simulink model "pha_0_5_servovalve"  (R2023a)
settings: Solver=VariableStepAuto  StartTime=0.0  StopTime=15  RelTol=1e-3
libraries: fl_lib x82, SimscapeFluids_lib x26, nesl_utility x8
(part 2 of 2)

== system pha_0_5_servovalve/Servovalve1/Nozzle B ==
  Nozzle B : SimscapeFluids_lib/Isothermal Liquid/Valves & Orifices/Orifices/Orifice (IL)  Tag=Factory Generic  orifice_type=foundation.enum.constant_variable.variable  constant_orifice_spec=fluids.isothermal_liquid.valves_orifices.orifices.enum.constant_orifice_spec.area  variable_orifice_spec=1  orifice_area_constant=1e-3 m^2  p_diff_TLU_constant=[-4, -3, -2, -1, -.5, 0, .5, 1, 2, 3, 4] MPa  vol_flow_TLU_constant=[-2.44, -2.12, -1.68, -1.22, -.84, 0, .85, 1.21, 1.7, 2.09, 2.41] .* 1e-3 m^3/s  S_min=2.9981e-07 m^2/mm  del_S=5.9981e-07 m^2/mm  open_orientation=-1  area_max=3.14 mm^2  area_leak=1e-9 m^2  S_TLU="-([  -0.002 0 0.005 0.015 ]) + 0.001*(0.3) m"  orifice_area_TLU="[  1e-12 4e-12 1e-05 1.02e-05 ] m^2"  area=inf m^2  Cd=0.7  Re_c=150  smoothing_factor=0  pressure_recovery=false  S_vol_flow_TLU="-([  -0.002 0 0.005 0.015 ]) + 0.001*(0.3) m"  p_diff_TLU="[  -5e+06 -2e+06 2e+06 5e+06 ] Pa"  vol_flow_TLU="[  -1e-12 -6e-14 6e+12 1e+11 ; -8e-08 -4e-08 4e+06 8e+06 ; -0.0025 -0.00103 0.001 0.0024 ; -0.00258 -0.001032 0.00106 0.00247 ; ] m^3/s"  enable_faults=simscape.enum.onoff.off  fault_action=fluids.enum.FaultOpening.Closed  external_fault=fluids.enum.FaultExternalTrigger.Off  temporal_fault=simscape.enum.onoff.off  fault_time=5 s  report_fault=simscape.enum.assert.action.none
      settings: InternalSimscapePortConfiguration="{\"Bottom\":[],\"Left\":[{\"id\":\"A\",\"label\":\"A\",\"type\":\"foundation.isothermal_liquid.isothermal_liquid\"},{\"id\":\"S\",\"label\":\"S\",\"type\":\"input\"}],\"Right\":[{\"id\":\"B\",\"label\":\"B\",\"type\":\"foundation.isothermal_liquid.isothermal_liquid\"}],\"Top\":[]}"
  S : PMIOPort  Side=Left
  A : PMIOPort  Port=2  Side=Left
  B : PMIOPort  Port=3  Side=Right
  connections:
  A/RConn1 -- Nozzle B/LConn1
  S/RConn1 -- Nozzle B/LConn2
  B/RConn1 -- Nozzle B/RConn1

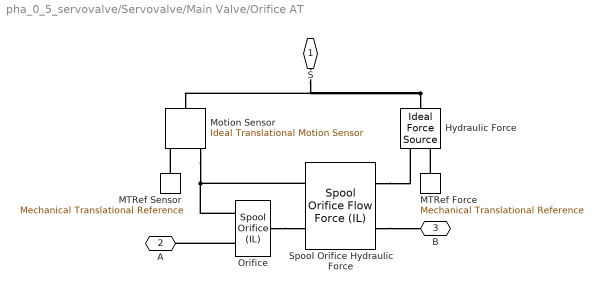
== system pha_0_5_servovalve/Servovalve/Main Valve/Orifice AT ==
  Hydraulic Force : fl_lib/Mechanical/Mechanical Sources/Ideal Force Source  Tag=Factory Generic
  MTRef Force : fl_lib/Mechanical/Translational Elements/Mechanical Translational Reference  Tag=Factory Generic
  MTRef Sensor : fl_lib/Mechanical/Translational Elements/Mechanical Translational Reference  Tag=Factory Generic
  Motion Sensor : fl_lib/Mechanical/Mechanical Sensors/Ideal Translational Motion Sensor  Tag=Factory Generic  reference=foundation.enum.MeasurementReference.difference  acceleration_port=false  velocity_port=true  position_port=true  offset=0 m
  Orifice : SimscapeFluids_lib/Isothermal Liquid/Valves & Orifices/Orifices/Spool Orifice (IL)  Tag=Factory Generic  orifice_spec=2  diameter_hole=5e-3 m  num_hole=6  width=24.5 mm  del_S_max=1 m  S_min=0.01 mm  open_orientation=-1  flow_force_spec=false  clearance=1e-5 m  area_leak=1e-9 m^2  area=inf m^2  Cd=0.7  Re_c=150  smoothing_factor=0  pressure_recovery=false
      settings: InternalSimscapePortConfiguration="{\"Bottom\":[],\"Left\":[{\"id\":\"S\",\"label\":\"S\",\"type\":\"input\"},{\"id\":\"A\",\"label\":\"A\",\"type\":\"foundation.isothermal_liquid.isothermal_liquid\"}],\"Right\":[{\"id\":\"B\",\"label\":\"B\",\"type\":\"foundation.isothermal_liquid.isothermal_liquid\"}],\"Top\":[]}"
  Spool Orifice Hydraulic Force : SimscapeFluids_lib/Isothermal Liquid/Valves & Orifices/Valve Actuators & Forces/Spool Orifice Flow Force (IL)  orifice_spec=2  diameter_hole=0.005 m  num_hole=4  width=24.5 mm  del_S_max=1 m  S_min=0.01 mm  open_orientation=-1  clearance=0.05 mm  area_leak=(24.5)*(0.05) mm^2  smoothing_factor=0
      settings: LibrarySourceBlock=SimscapeFluids_lib/Isothermal Liquid/Valves & Orifices/Valve Actuators & Forces/Spool Orifice Flow Force (IL)  InternalSimscapePortConfiguration="{\"Bottom\":[],\"Left\":[{\"id\":\"A\",\"label\":\"A\",\"type\":\"foundation.isothermal_liquid.isothermal_liquid\"},{\"id\":\"S\",\"label\":\"S\",\"type\":\"input\"}],\"Right\":[{\"id\":\"B\",\"label\":\"B\",\"type\":\"foundation.isothermal_liquid.isothermal_liquid\"},{\"id\":\"F\",\"label\":\"F\",\"type\":\"output\"}],\"Top\":[]}"
  S : PMIOPort  Side=Left
  A : PMIOPort  Port=2  Side=Left
  B : PMIOPort  Port=3  Side=Right
  connections:
  Motion Sensor/RConn3 -- Orifice/LConn1 -- Spool Orifice Hydraulic Force/LConn2
  Hydraulic Force/LConn1 -- Motion Sensor/LConn1 -- S/RConn1
  Orifice/RConn1 -- Spool Orifice Hydraulic Force/LConn1
  Orifice/LConn2 -- A/RConn1
  MTRef Force/LConn1 -- Hydraulic Force/RConn2
  MTRef Sensor/LConn1 -- Motion Sensor/RConn1
  Spool Orifice Hydraulic Force/RConn2 -- Hydraulic Force/RConn1
  Spool Orifice Hydraulic Force/RConn1 -- B/RConn1

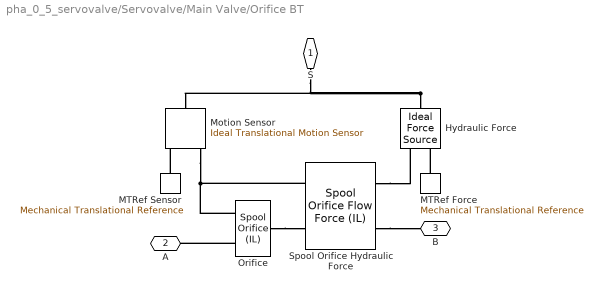
== system pha_0_5_servovalve/Servovalve/Main Valve/Orifice BT ==
  Hydraulic Force : fl_lib/Mechanical/Mechanical Sources/Ideal Force Source  Tag=Factory Generic
  MTRef Force : fl_lib/Mechanical/Translational Elements/Mechanical Translational Reference  Tag=Factory Generic
  MTRef Sensor : fl_lib/Mechanical/Translational Elements/Mechanical Translational Reference  Tag=Factory Generic
  Motion Sensor : fl_lib/Mechanical/Mechanical Sensors/Ideal Translational Motion Sensor  Tag=Factory Generic  reference=foundation.enum.MeasurementReference.difference  acceleration_port=false  velocity_port=true  position_port=true  offset=0 m
  Orifice : SimscapeFluids_lib/Isothermal Liquid/Valves & Orifices/Orifices/Spool Orifice (IL)  Tag=Factory Generic  orifice_spec=2  diameter_hole=5e-3 m  num_hole=6  width=24.5 mm  del_S_max=1 m  S_min=-(0.01) mm  open_orientation=1  flow_force_spec=false  clearance=1e-5 m  area_leak=1e-9 m^2  area=inf m^2  Cd=0.7  Re_c=150  smoothing_factor=0  pressure_recovery=false
      settings: InternalSimscapePortConfiguration="{\"Bottom\":[],\"Left\":[{\"id\":\"S\",\"label\":\"S\",\"type\":\"input\"},{\"id\":\"A\",\"label\":\"A\",\"type\":\"foundation.isothermal_liquid.isothermal_liquid\"}],\"Right\":[{\"id\":\"B\",\"label\":\"B\",\"type\":\"foundation.isothermal_liquid.isothermal_liquid\"}],\"Top\":[]}"
  Spool Orifice Hydraulic Force : SimscapeFluids_lib/Isothermal Liquid/Valves & Orifices/Valve Actuators & Forces/Spool Orifice Flow Force (IL)  orifice_spec=2  diameter_hole=0.005 m  num_hole=4  width=24.5 mm  del_S_max=1 m  S_min=-(0.01) mm  open_orientation=1  clearance=0.05 mm  area_leak=(24.5)*(0.05) mm^2  smoothing_factor=0
      settings: LibrarySourceBlock=SimscapeFluids_lib/Isothermal Liquid/Valves & Orifices/Valve Actuators & Forces/Spool Orifice Flow Force (IL)  InternalSimscapePortConfiguration="{\"Bottom\":[],\"Left\":[{\"id\":\"A\",\"label\":\"A\",\"type\":\"foundation.isothermal_liquid.isothermal_liquid\"},{\"id\":\"S\",\"label\":\"S\",\"type\":\"input\"}],\"Right\":[{\"id\":\"B\",\"label\":\"B\",\"type\":\"foundation.isothermal_liquid.isothermal_liquid\"},{\"id\":\"F\",\"label\":\"F\",\"type\":\"output\"}],\"Top\":[]}"
  S : PMIOPort  Side=Left
  A : PMIOPort  Port=2  Side=Left
  B : PMIOPort  Port=3  Side=Right
  connections:
  Motion Sensor/RConn3 -- Orifice/LConn1 -- Spool Orifice Hydraulic Force/LConn2
  Hydraulic Force/LConn1 -- Motion Sensor/LConn1 -- S/RConn1
  MTRef Sensor/LConn1 -- Motion Sensor/RConn1
  Orifice/LConn2 -- A/RConn1
  MTRef Force/LConn1 -- Hydraulic Force/RConn2
  Spool Orifice Hydraulic Force/RConn1 -- B/RConn1
  Spool Orifice Hydraulic Force/RConn2 -- Hydraulic Force/RConn1
  Orifice/RConn1 -- Spool Orifice Hydraulic Force/LConn1

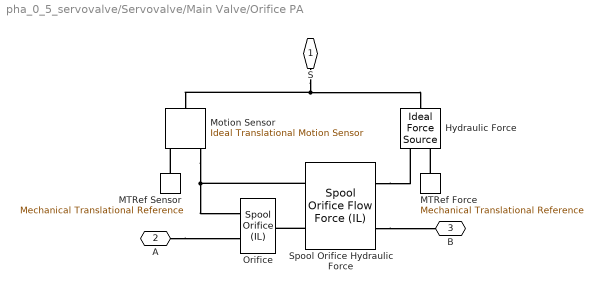
== system pha_0_5_servovalve/Servovalve/Main Valve/Orifice PA ==
  Hydraulic Force : fl_lib/Mechanical/Mechanical Sources/Ideal Force Source  Tag=Factory Generic
  MTRef Force : fl_lib/Mechanical/Translational Elements/Mechanical Translational Reference  Tag=Factory Generic
  MTRef Sensor : fl_lib/Mechanical/Translational Elements/Mechanical Translational Reference  Tag=Factory Generic
  Motion Sensor : fl_lib/Mechanical/Mechanical Sensors/Ideal Translational Motion Sensor  Tag=Factory Generic  reference=foundation.enum.MeasurementReference.difference  acceleration_port=false  velocity_port=true  position_port=true  offset=0 m
  Orifice : SimscapeFluids_lib/Isothermal Liquid/Valves & Orifices/Orifices/Spool Orifice (IL)  Tag=Factory Generic  orifice_spec=2  diameter_hole=5e-3 m  num_hole=6  width=24.5 mm  del_S_max=1 m  S_min=-(0.01) mm  open_orientation=1  flow_force_spec=false  clearance=1e-5 m  area_leak=1e-9 m^2  area=inf m^2  Cd=0.7  Re_c=150  smoothing_factor=0  pressure_recovery=false
      settings: InternalSimscapePortConfiguration="{\"Bottom\":[],\"Left\":[{\"id\":\"S\",\"label\":\"S\",\"type\":\"input\"},{\"id\":\"A\",\"label\":\"A\",\"type\":\"foundation.isothermal_liquid.isothermal_liquid\"}],\"Right\":[{\"id\":\"B\",\"label\":\"B\",\"type\":\"foundation.isothermal_liquid.isothermal_liquid\"}],\"Top\":[]}"
  Spool Orifice Hydraulic Force : SimscapeFluids_lib/Isothermal Liquid/Valves & Orifices/Valve Actuators & Forces/Spool Orifice Flow Force (IL)  orifice_spec=2  diameter_hole=0.005 m  num_hole=4  width=24.5 mm  del_S_max=1 m  S_min=-(0.01) mm  open_orientation=1  clearance=0.05 mm  area_leak=(24.5)*(0.05) mm^2  smoothing_factor=0
      settings: LibrarySourceBlock=SimscapeFluids_lib/Isothermal Liquid/Valves & Orifices/Valve Actuators & Forces/Spool Orifice Flow Force (IL)  InternalSimscapePortConfiguration="{\"Bottom\":[],\"Left\":[{\"id\":\"A\",\"label\":\"A\",\"type\":\"foundation.isothermal_liquid.isothermal_liquid\"},{\"id\":\"S\",\"label\":\"S\",\"type\":\"input\"}],\"Right\":[{\"id\":\"B\",\"label\":\"B\",\"type\":\"foundation.isothermal_liquid.isothermal_liquid\"},{\"id\":\"F\",\"label\":\"F\",\"type\":\"output\"}],\"Top\":[]}"
  S : PMIOPort  Side=Left
  A : PMIOPort  Port=2  Side=Left
  B : PMIOPort  Port=3  Side=Right
  connections:
  Spool Orifice Hydraulic Force/RConn2 -- Hydraulic Force/RConn1
  Spool Orifice Hydraulic Force/LConn1 -- Orifice/RConn1
  A/RConn1 -- Orifice/LConn2
  Spool Orifice Hydraulic Force/RConn1 -- B/RConn1
  Spool Orifice Hydraulic Force/LConn2 -- Motion Sensor/RConn3 -- Orifice/LConn1
  MTRef Sensor/LConn1 -- Motion Sensor/RConn1
  MTRef Force/LConn1 -- Hydraulic Force/RConn2
  S/RConn1 -- Motion Sensor/LConn1 -- Hydraulic Force/LConn1

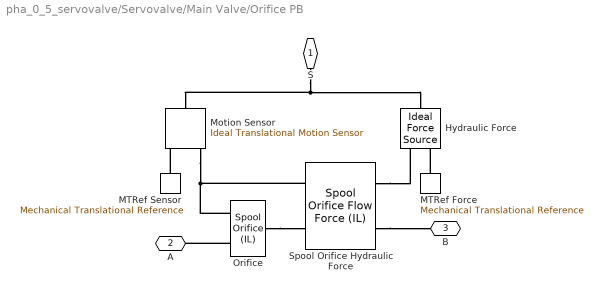
== system pha_0_5_servovalve/Servovalve/Main Valve/Orifice PB ==
  Hydraulic Force : fl_lib/Mechanical/Mechanical Sources/Ideal Force Source  Tag=Factory Generic
  MTRef Force : fl_lib/Mechanical/Translational Elements/Mechanical Translational Reference  Tag=Factory Generic
  MTRef Sensor : fl_lib/Mechanical/Translational Elements/Mechanical Translational Reference  Tag=Factory Generic
  Motion Sensor : fl_lib/Mechanical/Mechanical Sensors/Ideal Translational Motion Sensor  Tag=Factory Generic  reference=foundation.enum.MeasurementReference.difference  acceleration_port=false  velocity_port=true  position_port=true  offset=0 m
  Orifice : SimscapeFluids_lib/Isothermal Liquid/Valves & Orifices/Orifices/Spool Orifice (IL)  Tag=Factory Generic  orifice_spec=2  diameter_hole=5e-3 m  num_hole=6  width=24.5 mm  del_S_max=1 m  S_min=0.01 mm  open_orientation=-1  flow_force_spec=false  clearance=1e-5 m  area_leak=1e-9 m^2  area=inf m^2  Cd=0.7  Re_c=150  smoothing_factor=0  pressure_recovery=false
      settings: InternalSimscapePortConfiguration="{\"Bottom\":[],\"Left\":[{\"id\":\"S\",\"label\":\"S\",\"type\":\"input\"},{\"id\":\"A\",\"label\":\"A\",\"type\":\"foundation.isothermal_liquid.isothermal_liquid\"}],\"Right\":[{\"id\":\"B\",\"label\":\"B\",\"type\":\"foundation.isothermal_liquid.isothermal_liquid\"}],\"Top\":[]}"
  Spool Orifice Hydraulic Force : SimscapeFluids_lib/Isothermal Liquid/Valves & Orifices/Valve Actuators & Forces/Spool Orifice Flow Force (IL)  orifice_spec=2  diameter_hole=0.005 m  num_hole=4  width=24.5 mm  del_S_max=1 m  S_min=0.01 mm  open_orientation=-1  clearance=0.05 mm  area_leak=(24.5)*(0.05) mm^2  smoothing_factor=0
      settings: LibrarySourceBlock=SimscapeFluids_lib/Isothermal Liquid/Valves & Orifices/Valve Actuators & Forces/Spool Orifice Flow Force (IL)  InternalSimscapePortConfiguration="{\"Bottom\":[],\"Left\":[{\"id\":\"A\",\"label\":\"A\",\"type\":\"foundation.isothermal_liquid.isothermal_liquid\"},{\"id\":\"S\",\"label\":\"S\",\"type\":\"input\"}],\"Right\":[{\"id\":\"B\",\"label\":\"B\",\"type\":\"foundation.isothermal_liquid.isothermal_liquid\"},{\"id\":\"F\",\"label\":\"F\",\"type\":\"output\"}],\"Top\":[]}"
  S : PMIOPort  Side=Left
  A : PMIOPort  Port=2  Side=Left
  B : PMIOPort  Port=3  Side=Right
  connections:
  Motion Sensor/RConn3 -- Orifice/LConn1 -- Spool Orifice Hydraulic Force/LConn2
  S/RConn1 -- Motion Sensor/LConn1 -- Hydraulic Force/LConn1
  Spool Orifice Hydraulic Force/RConn2 -- Hydraulic Force/RConn1
  Orifice/LConn2 -- A/RConn1
  MTRef Force/LConn1 -- Hydraulic Force/RConn2
  MTRef Sensor/LConn1 -- Motion Sensor/RConn1
  Orifice/RConn1 -- Spool Orifice Hydraulic Force/LConn1
  Spool Orifice Hydraulic Force/RConn1 -- B/RConn1

== system pha_0_5_servovalve/Servovalve/Main Valve/Spool Side A ==
  Spool Side A : fl_lib/Isothermal Liquid/Elements/Translational Mechanical Converter (IL)  Tag=Factory Generic  mech_orientation=1  displacement_spec=foundation.enum.DisplacementSpec.Calculate  x0=0 m  interface_area=78 mm^2  dead_volume=1e-4 m^3  pressure_spec=1  environment_pressure=0.101325 MPa  dynamic_compressibility=0  p0=0 + 101325 Pa
      settings: LibrarySourceBlock=fl_lib/Isothermal Liquid/Elements/Translational Mechanical Converter (IL)  InternalSimscapePortConfiguration="{\"Bottom\":[],\"Left\":[{\"id\":\"A\",\"label\":\"A\",\"type\":\"foundation.isothermal_liquid.isothermal_liquid\"},{\"id\":\"C\",\"label\":\"C\",\"type\":\"foundation.mechanical.translational.translational\"}],\"Right\":[{\"id\":\"R\",\"label\":\"R\",\"type\":\"foundation.mechanical.translational.translational\"}],\"Top\":[]}"
  C : PMIOPort  Side=Left
  R : PMIOPort  Port=2  Side=Right
  A : PMIOPort  Port=3  Side=Left
  connections:
  A/RConn1 -- Spool Side A/LConn1
  C/RConn1 -- Spool Side A/LConn2
  Spool Side A/RConn1 -- R/RConn1

== system pha_0_5_servovalve/Servovalve/Main Valve/Spool Side B ==
  Spool Side B : fl_lib/Isothermal Liquid/Elements/Translational Mechanical Converter (IL)  Tag=Factory Generic  mech_orientation=-1  displacement_spec=foundation.enum.DisplacementSpec.Calculate  x0=-(0) m  interface_area=78 mm^2  dead_volume=1e-4 m^3  pressure_spec=1  environment_pressure=0.101325 MPa  dynamic_compressibility=0  p0=0 + 101325 Pa
      settings: LibrarySourceBlock=fl_lib/Isothermal Liquid/Elements/Translational Mechanical Converter (IL)  InternalSimscapePortConfiguration="{\"Bottom\":[],\"Left\":[{\"id\":\"A\",\"label\":\"A\",\"type\":\"foundation.isothermal_liquid.isothermal_liquid\"},{\"id\":\"C\",\"label\":\"C\",\"type\":\"foundation.mechanical.translational.translational\"}],\"Right\":[{\"id\":\"R\",\"label\":\"R\",\"type\":\"foundation.mechanical.translational.translational\"}],\"Top\":[]}"
  C : PMIOPort  Side=Left
  R : PMIOPort  Port=2  Side=Right
  A : PMIOPort  Port=3  Side=Left
  connections:
  R/RConn1 -- Spool Side B/RConn1
  Spool Side B/LConn1 -- A/RConn1
  Spool Side B/LConn2 -- C/RConn1

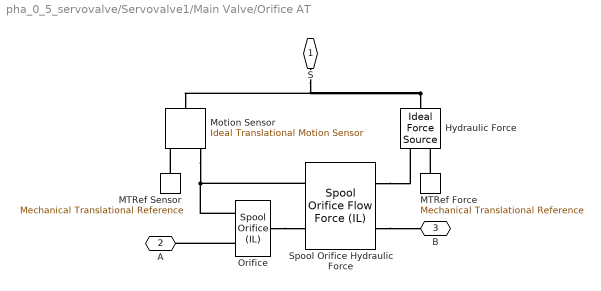
== system pha_0_5_servovalve/Servovalve1/Main Valve/Orifice AT ==
  Hydraulic Force : fl_lib/Mechanical/Mechanical Sources/Ideal Force Source  Tag=Factory Generic
  MTRef Force : fl_lib/Mechanical/Translational Elements/Mechanical Translational Reference  Tag=Factory Generic
  MTRef Sensor : fl_lib/Mechanical/Translational Elements/Mechanical Translational Reference  Tag=Factory Generic
  Motion Sensor : fl_lib/Mechanical/Mechanical Sensors/Ideal Translational Motion Sensor  Tag=Factory Generic  reference=foundation.enum.MeasurementReference.difference  acceleration_port=false  velocity_port=true  position_port=true  offset=0 m
  Orifice : SimscapeFluids_lib/Isothermal Liquid/Valves & Orifices/Orifices/Spool Orifice (IL)  Tag=Factory Generic  orifice_spec=2  diameter_hole=5e-3 m  num_hole=6  width=24.5 mm  del_S_max=1 m  S_min=0.01 mm  open_orientation=-1  flow_force_spec=false  clearance=1e-5 m  area_leak=1e-9 m^2  area=inf m^2  Cd=0.7  Re_c=150  smoothing_factor=0  pressure_recovery=false
      settings: InternalSimscapePortConfiguration="{\"Bottom\":[],\"Left\":[{\"id\":\"S\",\"label\":\"S\",\"type\":\"input\"},{\"id\":\"A\",\"label\":\"A\",\"type\":\"foundation.isothermal_liquid.isothermal_liquid\"}],\"Right\":[{\"id\":\"B\",\"label\":\"B\",\"type\":\"foundation.isothermal_liquid.isothermal_liquid\"}],\"Top\":[]}"
  Spool Orifice Hydraulic Force : SimscapeFluids_lib/Isothermal Liquid/Valves & Orifices/Valve Actuators & Forces/Spool Orifice Flow Force (IL)  orifice_spec=2  diameter_hole=0.005 m  num_hole=4  width=24.5 mm  del_S_max=1 m  S_min=0.01 mm  open_orientation=-1  clearance=0.05 mm  area_leak=(24.5)*(0.05) mm^2  smoothing_factor=0
      settings: LibrarySourceBlock=SimscapeFluids_lib/Isothermal Liquid/Valves & Orifices/Valve Actuators & Forces/Spool Orifice Flow Force (IL)  InternalSimscapePortConfiguration="{\"Bottom\":[],\"Left\":[{\"id\":\"A\",\"label\":\"A\",\"type\":\"foundation.isothermal_liquid.isothermal_liquid\"},{\"id\":\"S\",\"label\":\"S\",\"type\":\"input\"}],\"Right\":[{\"id\":\"B\",\"label\":\"B\",\"type\":\"foundation.isothermal_liquid.isothermal_liquid\"},{\"id\":\"F\",\"label\":\"F\",\"type\":\"output\"}],\"Top\":[]}"
  S : PMIOPort  Side=Left
  A : PMIOPort  Port=2  Side=Left
  B : PMIOPort  Port=3  Side=Right
  connections:
  Motion Sensor/RConn3 -- Orifice/LConn1 -- Spool Orifice Hydraulic Force/LConn2
  Hydraulic Force/LConn1 -- Motion Sensor/LConn1 -- S/RConn1
  Orifice/RConn1 -- Spool Orifice Hydraulic Force/LConn1
  Orifice/LConn2 -- A/RConn1
  MTRef Force/LConn1 -- Hydraulic Force/RConn2
  MTRef Sensor/LConn1 -- Motion Sensor/RConn1
  Spool Orifice Hydraulic Force/RConn2 -- Hydraulic Force/RConn1
  Spool Orifice Hydraulic Force/RConn1 -- B/RConn1

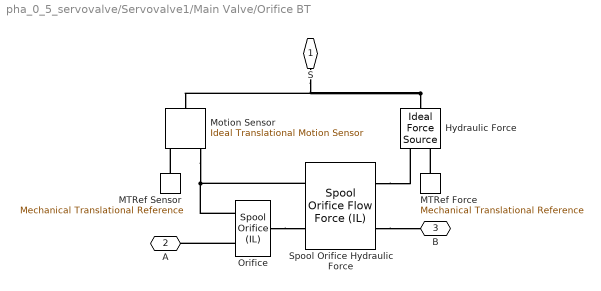
== system pha_0_5_servovalve/Servovalve1/Main Valve/Orifice BT ==
  Hydraulic Force : fl_lib/Mechanical/Mechanical Sources/Ideal Force Source  Tag=Factory Generic
  MTRef Force : fl_lib/Mechanical/Translational Elements/Mechanical Translational Reference  Tag=Factory Generic
  MTRef Sensor : fl_lib/Mechanical/Translational Elements/Mechanical Translational Reference  Tag=Factory Generic
  Motion Sensor : fl_lib/Mechanical/Mechanical Sensors/Ideal Translational Motion Sensor  Tag=Factory Generic  reference=foundation.enum.MeasurementReference.difference  acceleration_port=false  velocity_port=true  position_port=true  offset=0 m
  Orifice : SimscapeFluids_lib/Isothermal Liquid/Valves & Orifices/Orifices/Spool Orifice (IL)  Tag=Factory Generic  orifice_spec=2  diameter_hole=5e-3 m  num_hole=6  width=24.5 mm  del_S_max=1 m  S_min=-(0.01) mm  open_orientation=1  flow_force_spec=false  clearance=1e-5 m  area_leak=1e-9 m^2  area=inf m^2  Cd=0.7  Re_c=150  smoothing_factor=0  pressure_recovery=false
      settings: InternalSimscapePortConfiguration="{\"Bottom\":[],\"Left\":[{\"id\":\"S\",\"label\":\"S\",\"type\":\"input\"},{\"id\":\"A\",\"label\":\"A\",\"type\":\"foundation.isothermal_liquid.isothermal_liquid\"}],\"Right\":[{\"id\":\"B\",\"label\":\"B\",\"type\":\"foundation.isothermal_liquid.isothermal_liquid\"}],\"Top\":[]}"
  Spool Orifice Hydraulic Force : SimscapeFluids_lib/Isothermal Liquid/Valves & Orifices/Valve Actuators & Forces/Spool Orifice Flow Force (IL)  orifice_spec=2  diameter_hole=0.005 m  num_hole=4  width=24.5 mm  del_S_max=1 m  S_min=-(0.01) mm  open_orientation=1  clearance=0.05 mm  area_leak=(24.5)*(0.05) mm^2  smoothing_factor=0
      settings: LibrarySourceBlock=SimscapeFluids_lib/Isothermal Liquid/Valves & Orifices/Valve Actuators & Forces/Spool Orifice Flow Force (IL)  InternalSimscapePortConfiguration="{\"Bottom\":[],\"Left\":[{\"id\":\"A\",\"label\":\"A\",\"type\":\"foundation.isothermal_liquid.isothermal_liquid\"},{\"id\":\"S\",\"label\":\"S\",\"type\":\"input\"}],\"Right\":[{\"id\":\"B\",\"label\":\"B\",\"type\":\"foundation.isothermal_liquid.isothermal_liquid\"},{\"id\":\"F\",\"label\":\"F\",\"type\":\"output\"}],\"Top\":[]}"
  S : PMIOPort  Side=Left
  A : PMIOPort  Port=2  Side=Left
  B : PMIOPort  Port=3  Side=Right
  connections:
  Motion Sensor/RConn3 -- Orifice/LConn1 -- Spool Orifice Hydraulic Force/LConn2
  Hydraulic Force/LConn1 -- Motion Sensor/LConn1 -- S/RConn1
  MTRef Sensor/LConn1 -- Motion Sensor/RConn1
  Orifice/LConn2 -- A/RConn1
  MTRef Force/LConn1 -- Hydraulic Force/RConn2
  Spool Orifice Hydraulic Force/RConn1 -- B/RConn1
  Spool Orifice Hydraulic Force/RConn2 -- Hydraulic Force/RConn1
  Orifice/RConn1 -- Spool Orifice Hydraulic Force/LConn1

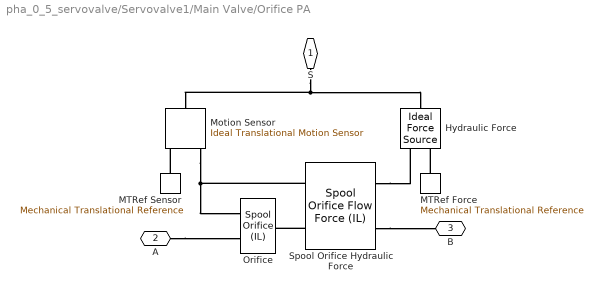
== system pha_0_5_servovalve/Servovalve1/Main Valve/Orifice PA ==
  Hydraulic Force : fl_lib/Mechanical/Mechanical Sources/Ideal Force Source  Tag=Factory Generic
  MTRef Force : fl_lib/Mechanical/Translational Elements/Mechanical Translational Reference  Tag=Factory Generic
  MTRef Sensor : fl_lib/Mechanical/Translational Elements/Mechanical Translational Reference  Tag=Factory Generic
  Motion Sensor : fl_lib/Mechanical/Mechanical Sensors/Ideal Translational Motion Sensor  Tag=Factory Generic  reference=foundation.enum.MeasurementReference.difference  acceleration_port=false  velocity_port=true  position_port=true  offset=0 m
  Orifice : SimscapeFluids_lib/Isothermal Liquid/Valves & Orifices/Orifices/Spool Orifice (IL)  Tag=Factory Generic  orifice_spec=2  diameter_hole=5e-3 m  num_hole=6  width=24.5 mm  del_S_max=1 m  S_min=-(0.01) mm  open_orientation=1  flow_force_spec=false  clearance=1e-5 m  area_leak=1e-9 m^2  area=inf m^2  Cd=0.7  Re_c=150  smoothing_factor=0  pressure_recovery=false
      settings: InternalSimscapePortConfiguration="{\"Bottom\":[],\"Left\":[{\"id\":\"S\",\"label\":\"S\",\"type\":\"input\"},{\"id\":\"A\",\"label\":\"A\",\"type\":\"foundation.isothermal_liquid.isothermal_liquid\"}],\"Right\":[{\"id\":\"B\",\"label\":\"B\",\"type\":\"foundation.isothermal_liquid.isothermal_liquid\"}],\"Top\":[]}"
  Spool Orifice Hydraulic Force : SimscapeFluids_lib/Isothermal Liquid/Valves & Orifices/Valve Actuators & Forces/Spool Orifice Flow Force (IL)  orifice_spec=2  diameter_hole=0.005 m  num_hole=4  width=24.5 mm  del_S_max=1 m  S_min=-(0.01) mm  open_orientation=1  clearance=0.05 mm  area_leak=(24.5)*(0.05) mm^2  smoothing_factor=0
      settings: LibrarySourceBlock=SimscapeFluids_lib/Isothermal Liquid/Valves & Orifices/Valve Actuators & Forces/Spool Orifice Flow Force (IL)  InternalSimscapePortConfiguration="{\"Bottom\":[],\"Left\":[{\"id\":\"A\",\"label\":\"A\",\"type\":\"foundation.isothermal_liquid.isothermal_liquid\"},{\"id\":\"S\",\"label\":\"S\",\"type\":\"input\"}],\"Right\":[{\"id\":\"B\",\"label\":\"B\",\"type\":\"foundation.isothermal_liquid.isothermal_liquid\"},{\"id\":\"F\",\"label\":\"F\",\"type\":\"output\"}],\"Top\":[]}"
  S : PMIOPort  Side=Left
  A : PMIOPort  Port=2  Side=Left
  B : PMIOPort  Port=3  Side=Right
  connections:
  Spool Orifice Hydraulic Force/RConn2 -- Hydraulic Force/RConn1
  Spool Orifice Hydraulic Force/LConn1 -- Orifice/RConn1
  A/RConn1 -- Orifice/LConn2
  Spool Orifice Hydraulic Force/RConn1 -- B/RConn1
  Spool Orifice Hydraulic Force/LConn2 -- Motion Sensor/RConn3 -- Orifice/LConn1
  MTRef Sensor/LConn1 -- Motion Sensor/RConn1
  MTRef Force/LConn1 -- Hydraulic Force/RConn2
  S/RConn1 -- Motion Sensor/LConn1 -- Hydraulic Force/LConn1

== system pha_0_5_servovalve/Servovalve1/Main Valve/Orifice PB ==
  Hydraulic Force : fl_lib/Mechanical/Mechanical Sources/Ideal Force Source  Tag=Factory Generic
  MTRef Force : fl_lib/Mechanical/Translational Elements/Mechanical Translational Reference  Tag=Factory Generic
  MTRef Sensor : fl_lib/Mechanical/Translational Elements/Mechanical Translational Reference  Tag=Factory Generic
  Motion Sensor : fl_lib/Mechanical/Mechanical Sensors/Ideal Translational Motion Sensor  Tag=Factory Generic  reference=foundation.enum.MeasurementReference.difference  acceleration_port=false  velocity_port=true  position_port=true  offset=0 m
  Orifice : SimscapeFluids_lib/Isothermal Liquid/Valves & Orifices/Orifices/Spool Orifice (IL)  Tag=Factory Generic  orifice_spec=2  diameter_hole=5e-3 m  num_hole=6  width=24.5 mm  del_S_max=1 m  S_min=0.01 mm  open_orientation=-1  flow_force_spec=false  clearance=1e-5 m  area_leak=1e-9 m^2  area=inf m^2  Cd=0.7  Re_c=150  smoothing_factor=0  pressure_recovery=false
      settings: InternalSimscapePortConfiguration="{\"Bottom\":[],\"Left\":[{\"id\":\"S\",\"label\":\"S\",\"type\":\"input\"},{\"id\":\"A\",\"label\":\"A\",\"type\":\"foundation.isothermal_liquid.isothermal_liquid\"}],\"Right\":[{\"id\":\"B\",\"label\":\"B\",\"type\":\"foundation.isothermal_liquid.isothermal_liquid\"}],\"Top\":[]}"
  Spool Orifice Hydraulic Force : SimscapeFluids_lib/Isothermal Liquid/Valves & Orifices/Valve Actuators & Forces/Spool Orifice Flow Force (IL)  orifice_spec=2  diameter_hole=0.005 m  num_hole=4  width=24.5 mm  del_S_max=1 m  S_min=0.01 mm  open_orientation=-1  clearance=0.05 mm  area_leak=(24.5)*(0.05) mm^2  smoothing_factor=0
      settings: LibrarySourceBlock=SimscapeFluids_lib/Isothermal Liquid/Valves & Orifices/Valve Actuators & Forces/Spool Orifice Flow Force (IL)  InternalSimscapePortConfiguration="{\"Bottom\":[],\"Left\":[{\"id\":\"A\",\"label\":\"A\",\"type\":\"foundation.isothermal_liquid.isothermal_liquid\"},{\"id\":\"S\",\"label\":\"S\",\"type\":\"input\"}],\"Right\":[{\"id\":\"B\",\"label\":\"B\",\"type\":\"foundation.isothermal_liquid.isothermal_liquid\"},{\"id\":\"F\",\"label\":\"F\",\"type\":\"output\"}],\"Top\":[]}"
  S : PMIOPort  Side=Left
  A : PMIOPort  Port=2  Side=Left
  B : PMIOPort  Port=3  Side=Right
  connections:
  Motion Sensor/RConn3 -- Orifice/LConn1 -- Spool Orifice Hydraulic Force/LConn2
  S/RConn1 -- Motion Sensor/LConn1 -- Hydraulic Force/LConn1
  Spool Orifice Hydraulic Force/RConn2 -- Hydraulic Force/RConn1
  Orifice/LConn2 -- A/RConn1
  MTRef Force/LConn1 -- Hydraulic Force/RConn2
  MTRef Sensor/LConn1 -- Motion Sensor/RConn1
  Orifice/RConn1 -- Spool Orifice Hydraulic Force/LConn1
  Spool Orifice Hydraulic Force/RConn1 -- B/RConn1

== system pha_0_5_servovalve/Servovalve1/Main Valve/Spool Side A ==
  Spool Side A : fl_lib/Isothermal Liquid/Elements/Translational Mechanical Converter (IL)  Tag=Factory Generic  mech_orientation=1  displacement_spec=foundation.enum.DisplacementSpec.Calculate  x0=0 m  interface_area=78 mm^2  dead_volume=1e-4 m^3  pressure_spec=1  environment_pressure=0.101325 MPa  dynamic_compressibility=0  p0=0 + 101325 Pa
      settings: LibrarySourceBlock=fl_lib/Isothermal Liquid/Elements/Translational Mechanical Converter (IL)  InternalSimscapePortConfiguration="{\"Bottom\":[],\"Left\":[{\"id\":\"A\",\"label\":\"A\",\"type\":\"foundation.isothermal_liquid.isothermal_liquid\"},{\"id\":\"C\",\"label\":\"C\",\"type\":\"foundation.mechanical.translational.translational\"}],\"Right\":[{\"id\":\"R\",\"label\":\"R\",\"type\":\"foundation.mechanical.translational.translational\"}],\"Top\":[]}"
  C : PMIOPort  Side=Left
  R : PMIOPort  Port=2  Side=Right
  A : PMIOPort  Port=3  Side=Left
  connections:
  A/RConn1 -- Spool Side A/LConn1
  C/RConn1 -- Spool Side A/LConn2
  Spool Side A/RConn1 -- R/RConn1

== system pha_0_5_servovalve/Servovalve1/Main Valve/Spool Side B ==
  Spool Side B : fl_lib/Isothermal Liquid/Elements/Translational Mechanical Converter (IL)  Tag=Factory Generic  mech_orientation=-1  displacement_spec=foundation.enum.DisplacementSpec.Calculate  x0=-(0) m  interface_area=78 mm^2  dead_volume=1e-4 m^3  pressure_spec=1  environment_pressure=0.101325 MPa  dynamic_compressibility=0  p0=0 + 101325 Pa
      settings: LibrarySourceBlock=fl_lib/Isothermal Liquid/Elements/Translational Mechanical Converter (IL)  InternalSimscapePortConfiguration="{\"Bottom\":[],\"Left\":[{\"id\":\"A\",\"label\":\"A\",\"type\":\"foundation.isothermal_liquid.isothermal_liquid\"},{\"id\":\"C\",\"label\":\"C\",\"type\":\"foundation.mechanical.translational.translational\"}],\"Right\":[{\"id\":\"R\",\"label\":\"R\",\"type\":\"foundation.mechanical.translational.translational\"}],\"Top\":[]}"
  C : PMIOPort  Side=Left
  R : PMIOPort  Port=2  Side=Right
  A : PMIOPort  Port=3  Side=Left
  connections:
  R/RConn1 -- Spool Side B/RConn1
  Spool Side B/LConn1 -- A/RConn1
  Spool Side B/LConn2 -- C/RConn1
